simulink model "ret_n_controlado_3f"  (R2017a)
settings: Solver=VariableStepAuto  StartTime=0.0  StopTime=1/30  RelTol=1e-3
libraries: fl_lib x22, nesl_utility x12
settings Model: Creator=gabriel  LastModifiedBy=gabriel

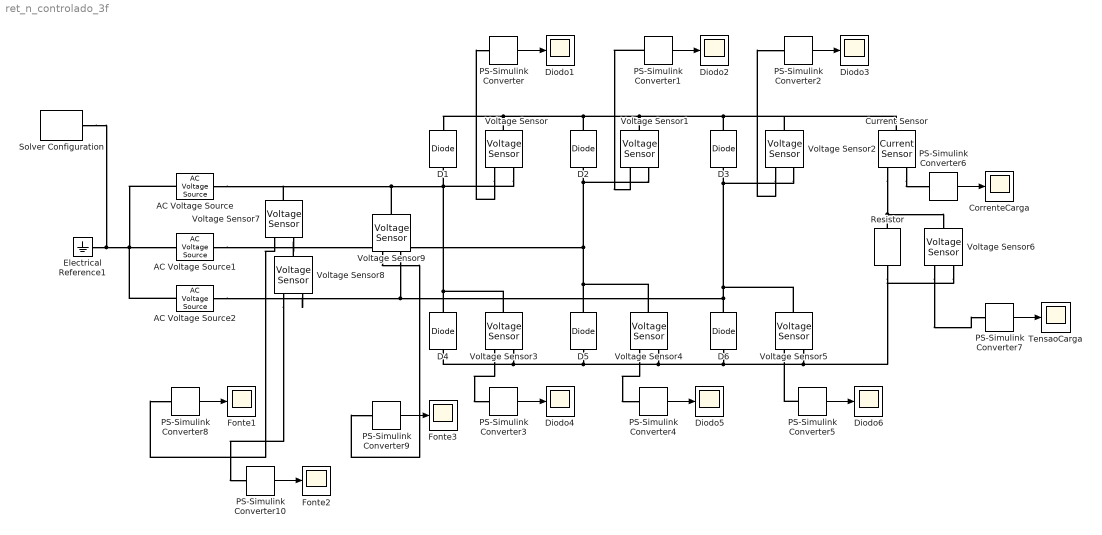
== system ret_n_controlado_3f ==
  AC Voltage Source : fl_lib/Electrical/Electrical Sources/AC Voltage Source  amp=130*sqrt(2) V  shift=0 deg  frequency=60 Hz  omega=0 rad/s
  AC Voltage Source1 : fl_lib/Electrical/Electrical Sources/AC Voltage Source  amp=130*sqrt(2) V  shift=120 deg  frequency=60 Hz  omega=0 rad/s
  AC Voltage Source2 : fl_lib/Electrical/Electrical Sources/AC Voltage Source  amp=130*sqrt(2) V  shift=240 deg  frequency=60 Hz  omega=0 rad/s
  CorrenteCarga : Scope
  Current Sensor : fl_lib/Electrical/Electrical Sensors/Current Sensor
  D{1..6} (6 alike) : fl_lib/Electrical/Electrical Elements/Diode  Vf=0.6 V  Ron=0.3 Ohm  Goff=1e-8 1/Ohm  i_specify=off  i_priority=None  i=0 A  i_nominal_specify=off  i_nominal_unit=A  i_nominal_value=1  v_specify=off  v_priority=None  v=0 V  v_nominal_specify=off  v_nominal_unit=V  v_nominal_value=1
  Diodo{1..6} (6 alike) : Scope
  Electrical Reference1 : fl_lib/Electrical/Electrical Elements/Electrical Reference
  Fonte1 : Scope
  Fonte2 : Scope
  Fonte3 : Scope
  PS-Simulink Converter{,1..10} (11 alike) : nesl_utility/PS-Simulink Converter  PhysicalDomain=network_engine_domain  SubClassName=ps_output  LeftPortType=input  RightPortType=output  PseudoPeriodic=off  Frequencies=[]  Unit=1  AffineConversion=off
  Resistor : fl_lib/Electrical/Electrical Elements/Resistor  R=65.7+65.5 Ohm  i_specify=off  i_priority=None  i=0 A  i_nominal_specify=off  i_nominal_unit=A  i_nominal_value=1  v_specify=off  v_priority=None  v=0 V  v_nominal_specify=off  v_nominal_unit=V  v_nominal_value=1
  Solver Configuration : nesl_utility/Solver Configuration  PhysicalDomain=network_engine_domain  SubClassName=solver  LeftPortType=input  RightPortType=generic  Accelerate=off  Tones=[]  Harmonics=[]  SimulateNoise=off  Profile=off  UseLocalSampling=off  EnableSwitchedLinearOptims=on  FrequencyDomain=off  UseCCode=off  RelTol=0.001  AbsTol=1e-06  MinStep=1e-09  ToWorkspace=off  RevertToSquareIcSolve=off  NumHomotopyIterations=100  PhasorMode=off  PhasorModeNumHarmonics=1  OverrideAbsTol=off  DoDC=off  ResidualTolerance=1e-09  UseLocalSolver=off  LocalSolverChoice=NE_BACKWARD_EULER_ADVANCER  LocalSolverSampleTime=0.001  DoFixedCost=off  MaxNonlinIter=3  MaxModeIter=2  LinearAlgebra=Sparse  DelaysMemoryBudget=1024  AutomaticFiltering=on  FilteringTimeConstant=0.001
  TensaoCarga : Scope
  Voltage Sensor{,1..9} (10 alike) : fl_lib/Electrical/Electrical Sensors/Voltage Sensor
  wires:
  PS-Simulink Converter/1 -> Diodo1/1
  PS-Simulink Converter1/1 -> Diodo2/1
  PS-Simulink Converter2/1 -> Diodo3/1
  PS-Simulink Converter3/1 -> Diodo4/1
  PS-Simulink Converter4/1 -> Diodo5/1
  PS-Simulink Converter5/1 -> Diodo6/1
  PS-Simulink Converter6/1 -> CorrenteCarga/1
  PS-Simulink Converter7/1 -> TensaoCarga/1
  PS-Simulink Converter8/1 -> Fonte1/1
  PS-Simulink Converter9/1 -> Fonte3/1
  PS-Simulink Converter10/1 -> Fonte2/1
  connections:
  D5/RConn1 -- Voltage Sensor4/LConn1 -- Voltage Sensor8/LConn1 -- Voltage Sensor7/RConn2 -- AC Voltage Source1/LConn1 -- Voltage Sensor1/RConn2 -- D2/LConn1
  D4/RConn1 -- Voltage Sensor3/LConn1 -- Voltage Sensor9/LConn1 -- Voltage Sensor7/LConn1 -- AC Voltage Source/LConn1 -- Voltage Sensor/RConn2 -- D1/LConn1
  D6/RConn1 -- Voltage Sensor9/RConn2 -- Voltage Sensor8/RConn2 -- AC Voltage Source2/LConn1 -- Voltage Sensor5/LConn1 -- Voltage Sensor2/RConn2 -- D3/LConn1
  D6/LConn1 -- Voltage Sensor6/RConn2 -- Resistor/RConn1 -- Voltage Sensor5/RConn2 -- Voltage Sensor4/RConn2 -- D5/LConn1 -- Voltage Sensor3/RConn2 -- D4/LConn1
  D3/RConn1 -- Current Sensor/LConn1 -- Voltage Sensor2/LConn1 -- Voltage Sensor1/LConn1 -- D2/RConn1 -- Voltage Sensor/LConn1 -- D1/RConn1
  Electrical Reference1/LConn1 -- Solver Configuration/RConn1 -- AC Voltage Source/RConn1 -- AC Voltage Source2/RConn1 -- AC Voltage Source1/RConn1
  Resistor/LConn1 -- Current Sensor/RConn2 -- Voltage Sensor6/LConn1
  Voltage Sensor/RConn1 -- PS-Simulink Converter/LConn1
  PS-Simulink Converter1/LConn1 -- Voltage Sensor1/RConn1
  Voltage Sensor2/RConn1 -- PS-Simulink Converter2/LConn1
  Voltage Sensor3/RConn1 -- PS-Simulink Converter3/LConn1
  Voltage Sensor4/RConn1 -- PS-Simulink Converter4/LConn1
  PS-Simulink Converter5/LConn1 -- Voltage Sensor5/RConn1
  Current Sensor/RConn1 -- PS-Simulink Converter6/LConn1
  Voltage Sensor6/RConn1 -- PS-Simulink Converter7/LConn1
  Voltage Sensor7/RConn1 -- PS-Simulink Converter8/LConn1
  Voltage Sensor8/RConn1 -- PS-Simulink Converter10/LConn1
  Voltage Sensor9/RConn1 -- PS-Simulink Converter9/LConn1
